simulink model "test_rx"  (Simulink 7.6)
settings: Solver=FixedStepDiscrete  StartTime=0.0  StopTime=2  FixedStep=1  RelTol=1e-3
libraries: simulink x20
settings Model: Creator=jordan  LastModifiedBy=jordan
settings DataIOCC: LimitDataPoints=off  SaveOutput=off  SignalLogging=off  DSMLogging=off  SaveTime=off
settings OptimizationCC: BlockReduction=off  ConditionallyExecuteInputs=off  InlineParams=on

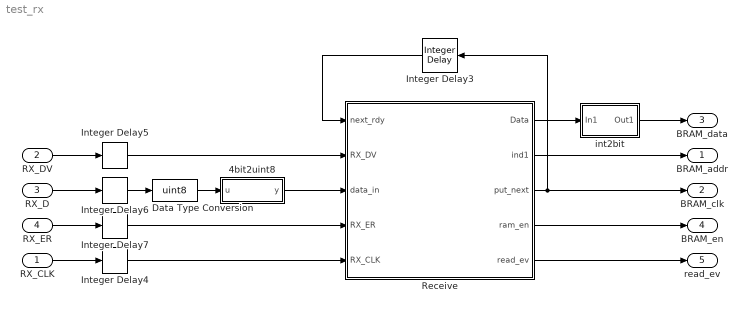
== system test_rx ==
  RX_CLK : Inport  OutDataTypeStr=boolean
  RX_DV : Inport  Port=2  OutDataTypeStr=boolean
  RX_D : Inport  Port=3  OutDataTypeStr=boolean  PortDimensions=4
  RX_ER : Inport  Port=4  OutDataTypeStr=boolean  PortDimensions=1
  4bit2uint8 : Stateflow chart  TreatAsAtomicUnit=on
  Data Type Conversion : DataTypeConversion  OutDataTypeStr=uint8
  Integer Delay{3..7} (5 alike) : simulink/Discrete/Integer Delay  NumDelays=1  vinit=0.0  samptime=-1
  Receive : Stateflow chart  TreatAsAtomicUnit=on
  int2bit : Subsystem
  BRAM_addr : Outport
  BRAM_clk : Outport  Port=2
  BRAM_data : Outport  Port=3
  BRAM_en : Outport  Port=4
  read_ev : Outport  Port=5
  wires:
  Receive/2(ind1) -> BRAM_addr/1
  Receive/3(put_next) -> Integer Delay3/1, BRAM_clk/1
  RX_CLK/1 -> Integer Delay4/1
  RX_DV/1 -> Integer Delay5/1
  RX_D/1 -> Integer Delay6/1
  RX_ER/1 -> Integer Delay7/1
  Receive/1(Data) -> int2bit/1(In1)
  Integer Delay4/1 -> Receive/5(RX_CLK)
  Integer Delay5/1 -> Receive/2(RX_DV)
  Integer Delay6/1 -> Data Type Conversion/1
  Integer Delay7/1 -> Receive/4(RX_ER)
  Integer Delay3/1 -> Receive/1(next_rdy)
  4bit2uint8/1(y) -> Receive/3(data_in)
  Data Type Conversion/1 -> 4bit2uint8/1(u)
  Receive/4(ram_en) -> BRAM_en/1
  Receive/5(read_ev) -> read_ev/1
  int2bit/1(Out1) -> BRAM_data/1

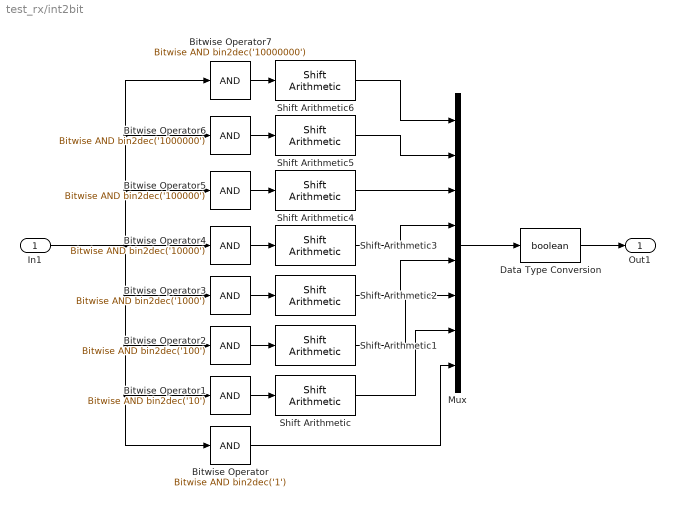
== system test_rx/int2bit ==
  In1 : Inport  OutDataTypeStr=uint8
  Bitwise Operator : simulink/Logic and Bit Operations/Bitwise Operator  logicop=AND  UseBitMask=on  BitMask=bin2dec('1')  BitMaskRealWorld=Stored Integer
  Bitwise Operator1 : simulink/Logic and Bit Operations/Bitwise Operator  logicop=AND  UseBitMask=on  BitMask=bin2dec('10')  BitMaskRealWorld=Stored Integer
  Bitwise Operator2 : simulink/Logic and Bit Operations/Bitwise Operator  logicop=AND  UseBitMask=on  BitMask=bin2dec('100')  BitMaskRealWorld=Stored Integer
  Bitwise Operator3 : simulink/Logic and Bit Operations/Bitwise Operator  logicop=AND  UseBitMask=on  BitMask=bin2dec('1000')  BitMaskRealWorld=Stored Integer
  Bitwise Operator4 : simulink/Logic and Bit Operations/Bitwise Operator  logicop=AND  UseBitMask=on  BitMask=bin2dec('10000')  BitMaskRealWorld=Stored Integer
  Bitwise Operator5 : simulink/Logic and Bit Operations/Bitwise Operator  logicop=AND  UseBitMask=on  BitMask=bin2dec('100000')  BitMaskRealWorld=Stored Integer
  Bitwise Operator6 : simulink/Logic and Bit Operations/Bitwise Operator  logicop=AND  UseBitMask=on  BitMask=bin2dec('1000000')  BitMaskRealWorld=Stored Integer
  Bitwise Operator7 : simulink/Logic and Bit Operations/Bitwise Operator  logicop=AND  UseBitMask=on  BitMask=bin2dec('10000000')  BitMaskRealWorld=Stored Integer
  Data Type Conversion : DataTypeConversion  OutDataTypeStr=boolean
  Mux : Mux  Inputs=8
  Shift Arithmetic : simulink/Logic and Bit Operations/Shift Arithmetic  SystemSampleTime=-1  nBitShiftRight=1  nBinPtShiftRight=0
  Shift Arithmetic1 : simulink/Logic and Bit Operations/Shift Arithmetic  SystemSampleTime=-1  nBitShiftRight=2  nBinPtShiftRight=0
  Shift Arithmetic2 : simulink/Logic and Bit Operations/Shift Arithmetic  SystemSampleTime=-1  nBitShiftRight=3  nBinPtShiftRight=0
  Shift Arithmetic3 : simulink/Logic and Bit Operations/Shift Arithmetic  SystemSampleTime=-1  nBitShiftRight=4  nBinPtShiftRight=0
  Shift Arithmetic4 : simulink/Logic and Bit Operations/Shift Arithmetic  SystemSampleTime=-1  nBitShiftRight=5  nBinPtShiftRight=0
  Shift Arithmetic5 : simulink/Logic and Bit Operations/Shift Arithmetic  SystemSampleTime=-1  nBitShiftRight=6  nBinPtShiftRight=0
  Shift Arithmetic6 : simulink/Logic and Bit Operations/Shift Arithmetic  SystemSampleTime=-1  nBitShiftRight=7  nBinPtShiftRight=0
  Out1 : Outport  InitialOutput=0
  wires:
  Data Type Conversion/1 -> Out1/1
  Mux/1 -> Data Type Conversion/1
  Bitwise Operator7/1 -> Shift Arithmetic6/1
  Bitwise Operator6/1 -> Shift Arithmetic5/1
  Bitwise Operator5/1 -> Shift Arithmetic4/1
  Bitwise Operator4/1 -> Shift Arithmetic3/1
  Bitwise Operator3/1 -> Shift Arithmetic2/1
  Bitwise Operator2/1 -> Shift Arithmetic1/1
  Bitwise Operator1/1 -> Shift Arithmetic/1
  In1/1 -> Bitwise Operator4/1, Bitwise Operator7/1, Bitwise Operator6/1, Bitwise Operator5/1, Bitwise Operator3/1, Bitwise Operator2/1, Bitwise Operator1/1, Bitwise Operator/1
  Shift Arithmetic6/1 -> Mux/1
  Shift Arithmetic5/1 -> Mux/2
  Shift Arithmetic4/1 -> Mux/3
  Shift Arithmetic3/1 -> Mux/4
  Shift Arithmetic2/1 -> Mux/5
  Shift Arithmetic1/1 -> Mux/6
  Shift Arithmetic/1 -> Mux/7
  Bitwise Operator/1 -> Mux/8

== matlab function 4bit2uint8 ==
  data: u input uint8 size=4; y output uint8
function y = fcn(u)
%#eml
y = uint8(bitor(bitor(bitor(u(1),bitshift(u(2),1)),bitshift(u(3),2)),bitshift(u(4),3)));

== stateflow chart Receive ==
  settings: executeAtInitialization=1
  state Wait1
  state Start_RX
  state Wait2
  state Error
  state Wait_low
  state Read
  state WriteRAM
  state Read_rdy
  state Read_rdy1
  (default) -> Start_RX
  (junction 19) -> Start_RX [order 2]
  (junction 19) -> (junction 21) [order 1] : [RX_DV==1]{
      | put_next=0;}
  (junction 23) -> Read [order 2]
  Read -> Wait1 : [RX_CLK==0]{
      | buf_rx=data_in;}
  Wait2 -> WriteRAM : [RX_CLK==0]{
      | buf1=data_in<<4;
      | buf_rx=buf_rx|buf1;
      | put_next=1;
      | ram_en=1;
      | Data=buf_rx;}
  Read_rdy -> Read_rdy1 : {read_ev=0;
      | Data=0;}
  WriteRAM -> (junction 22) : [next_rdy==1]{
      | put_next=0;
      | ram_en=0;}
  Wait_low -> (junction 19) : [RX_CLK==0]{
      | put_next=0;}
  (junction 20) -> Start_RX
  (junction 22) -> Read_rdy [order 2] : {Pack_on_line=0;
      | read_ev=1;
      | ind1=0;}
  Start_RX -> Wait_low : [RX_CLK==1]{put_next=0;}
  (junction 21) -> (junction 23) [order 2]
  Wait1 -> Wait2 : [RX_CLK==1]
  (junction 22) -> (junction 20) [order 1] : [ind1<64]{ind1++;}
  (junction 21) -> Error [order 1] : [RX_ER==1]
  Error -> Start_RX : [RX_DV==0]{
      | Pack_on_line=0;}
  (junction 23) -> Read [order 1] : [Pack_on_line==0]{
      | Pack_on_line=1;
      | put_next=0;
      | ind1=0;CRC=0;}
  Read_rdy1 -> (junction 20) : [RX_DV==0]
  data: Data output uint8 =0; ind1 output fixdt(0,11,0); CRC local uint32; put_next output boolean =0; next_rdy input boolean; buf_rx local uint8; buf_bit local boolean; gen_poly constant uint32 =79764919; buf32 local uint32; Pack_on_line local boolean =0; buf1 local uint8; RX_DV input boolean; data_in input uint8; RX_ER input boolean; RX_CLK input boolean; ram_en output boolean; read_ev output boolean
